simulink model "TorqueDistributionModel"  (Simulink 7.4)
settings: Solver=ode45  StartTime=0.0  StopTime=10.0  RelTol=1e-3
undefined symbols (not defined in the file or in its folder): F_bias, F_fl, F_flz, F_fr, F_frz, F_powertrain, F_rlz, F_rrz, sparse, speye, x1, x2
libraries: BLOM_Lib x16
settings Model: Creator=Kyle  LastModifiedBy=Kyle

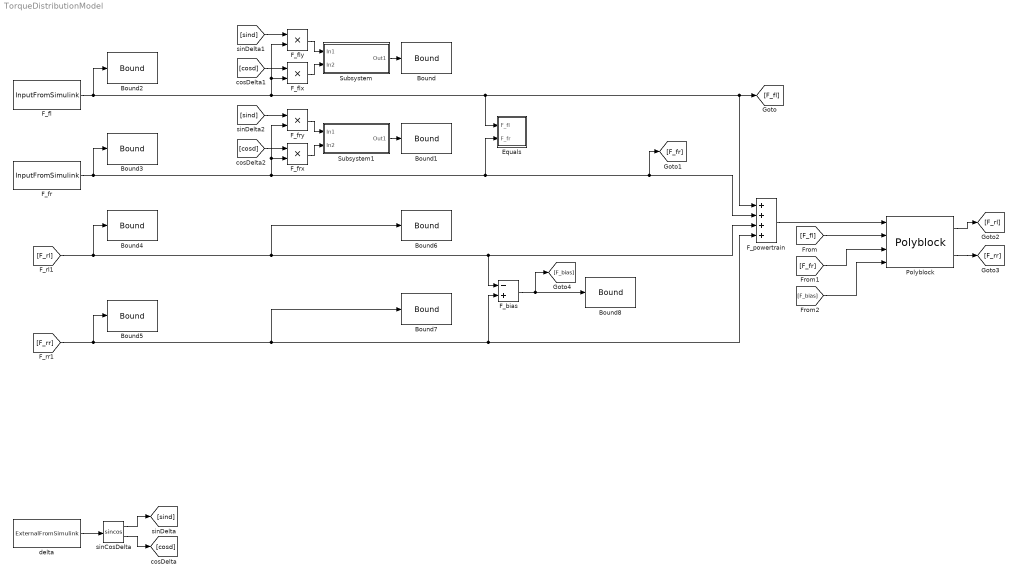
== system TorqueDistributionModel ==
  Bound : BLOM_Lib/Bound  SystemSampleTime=-1  ub=u*F_flz  lb=-inf  initial_step=on  intermediate_step=on  final_step=on
  Bound1 : BLOM_Lib/Bound  SystemSampleTime=-1  ub=u*F_frz  lb=-inf  initial_step=on  intermediate_step=on  final_step=on
  Bound2 : BLOM_Lib/Bound  SystemSampleTime=-1  ub=F_fl_max  lb=F_fl_min  initial_step=on  intermediate_step=on  final_step=on
  Bound3 : BLOM_Lib/Bound  SystemSampleTime=-1  ub=F_fr_max  lb=F_fr_min  initial_step=on  intermediate_step=on  final_step=on
  Bound4 : BLOM_Lib/Bound  SystemSampleTime=-1  ub=F_rl_max  lb=F_rl_min  initial_step=on  intermediate_step=on  final_step=on
  Bound5 : BLOM_Lib/Bound  SystemSampleTime=-1  ub=F_rr_max  lb=F_rr_min  initial_step=on  intermediate_step=on  final_step=on
  Bound6 : BLOM_Lib/Bound  SystemSampleTime=-1  ub=u*F_rlz  lb=-inf  initial_step=on  intermediate_step=on  final_step=on
  Bound7 : BLOM_Lib/Bound  SystemSampleTime=-1  ub=u*F_rrz  lb=-inf  initial_step=on  intermediate_step=on  final_step=on
  Bound8 : BLOM_Lib/Bound  SystemSampleTime=-1  ub=F_clutch_max  lb=-inf  initial_step=on  intermediate_step=on  final_step=on
  Equals : Subsystem
  F_bias : Sum  Inputs=-+  OutDataType=fixdt(1, 16)  OutScaling=2^-10
  F_fl : BLOM_Lib/InputFromSimulink  SystemSampleTime=-1  interpType=Zero-Order Hold
  F_flx : Product  OutDataType=fixdt(1, 16)  OutScaling=2^0  RndMeth=Zero
  F_fly : Product  OutDataType=fixdt(1, 16)  OutScaling=2^0  RndMeth=Zero
  F_fr : BLOM_Lib/InputFromSimulink  SystemSampleTime=-1  interpType=Zero-Order Hold
  F_frx : Product  OutDataType=fixdt(1, 16)  OutScaling=2^0  RndMeth=Zero
  F_fry : Product  OutDataType=fixdt(1, 16)  OutScaling=2^0  RndMeth=Zero
  F_powertrain : Sum  Inputs=4  OutDataType=fixdt(1, 16)  OutScaling=2^-10
  Polyblock : BLOM_Lib/Polyblock  SystemSampleTime=-1  P=speye(4)  K=sparse([.5 -.5 -.5 -.5; .5 -.5 -.5 .5])  inputs=F_powertrain,F_fl,F_fr,F_bias  inputScalar=on  outputScalar=on
  Subsystem : Subsystem
  Subsystem1 : Subsystem
  delta : BLOM_Lib/ExternalFromSimulink  SystemSampleTime=-1  interpType=Zero-Order Hold
  sinCosDelta : Trigonometry  Operator=sincos
  wires:
  F_fl/1 -> F_fly/2, F_flx/2, Equals/1(F_fl), F_powertrain/1, [F_fl], Bound2/1
  [F_rl] -> Bound4/1, Bound6/1, F_bias/1, F_powertrain/3
  [F_rr] -> Bound5/1, Bound7/1, F_bias/2, F_powertrain/4
  delta/1 -> sinCosDelta/1
  sinCosDelta/1 -> [sind]
  sinCosDelta/2 -> [cosd]
  F_fr/1 -> F_fry/2, F_frx/2, Equals/2(F_fr), F_powertrain/2, [F_fr], Bound3/1
  [cosd] -> F_frx/1
  [sind] -> F_fry/1
  [sind] -> F_fly/1
  [cosd] -> F_flx/1
  F_fly/1 -> Subsystem/1(In1)
  F_flx/1 -> Subsystem/2(In2)
  Subsystem/1(Out1) -> Bound/1
  Subsystem1/1(Out1) -> Bound1/1
  F_fry/1 -> Subsystem1/1(In1)
  F_frx/1 -> Subsystem1/2(In2)
  F_bias/1 -> Bound8/1, [F_bias]
  F_powertrain/1 -> Polyblock/1
  [F_fl] -> Polyblock/2
  [F_fr] -> Polyblock/3
  [F_bias] -> Polyblock/4
  Polyblock/1 -> [F_rl]
  Polyblock/2 -> [F_rr]

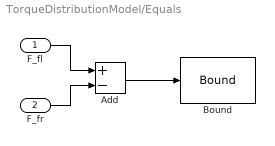
== system TorqueDistributionModel/Equals ==
  F_fl : Inport  OutDataType=fixdt(1, 16)  OutScaling=2^0
  F_fr : Inport  Port=2  OutDataType=fixdt(1, 16)  OutScaling=2^0
  Add : Sum  Inputs=+-  OutDataType=fixdt(1, 16)  OutScaling=2^-10
  Bound : BLOM_Lib/Bound  SystemSampleTime=-1  ub=0  lb=0  initial_step=on  intermediate_step=on  final_step=on
  wires:
  F_fl/1 -> Add/1
  F_fr/1 -> Add/2
  Add/1 -> Bound/1

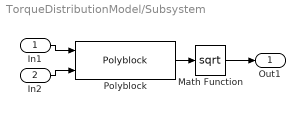
== system TorqueDistributionModel/Subsystem ==
  In1 : Inport  OutDataType=fixdt(1, 16)  OutScaling=2^0
  In2 : Inport  Port=2  OutDataType=fixdt(1, 16)  OutScaling=2^0
  Math Function : Math  Operator=sqrt  OutDataType=fixdt(1, 16)  OutScaling=2^0  SaturateOnIntegerOverflow=on
  Polyblock : BLOM_Lib/Polyblock  SystemSampleTime=-1  P=sparse([2 0; 0 2 ])  K=sparse([1 -1])  inputs=x1,x2  inputScalar=on  outputScalar=on
  Out1 : Outport  OutDataType=fixdt(1, 16)  OutScaling=2^0
  wires:
  In1/1 -> Polyblock/1
  In2/1 -> Polyblock/2
  Polyblock/1 -> Math Function/1
  Math Function/1 -> Out1/1

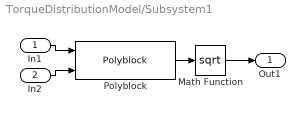
== system TorqueDistributionModel/Subsystem1 ==
  In1 : Inport  OutDataType=fixdt(1, 16)  OutScaling=2^0
  In2 : Inport  Port=2  OutDataType=fixdt(1, 16)  OutScaling=2^0
  Math Function : Math  Operator=sqrt  OutDataType=fixdt(1, 16)  OutScaling=2^0  SaturateOnIntegerOverflow=on
  Polyblock : BLOM_Lib/Polyblock  SystemSampleTime=-1  P=sparse([2 0; 0 2 ])  K=sparse([1 -1])  inputs=x1,x2  inputScalar=on  outputScalar=on
  Out1 : Outport  OutDataType=fixdt(1, 16)  OutScaling=2^0
  wires:
  In1/1 -> Polyblock/1
  In2/1 -> Polyblock/2
  Polyblock/1 -> Math Function/1
  Math Function/1 -> Out1/1
